simulink model "dss_test"  (Simulink 8.4)
settings: Solver=ode45  StartTime=0.0  StopTime=10.0  RelTol=1e-3
settings Model: Creator=arnaud  LastModifiedBy=arnaud

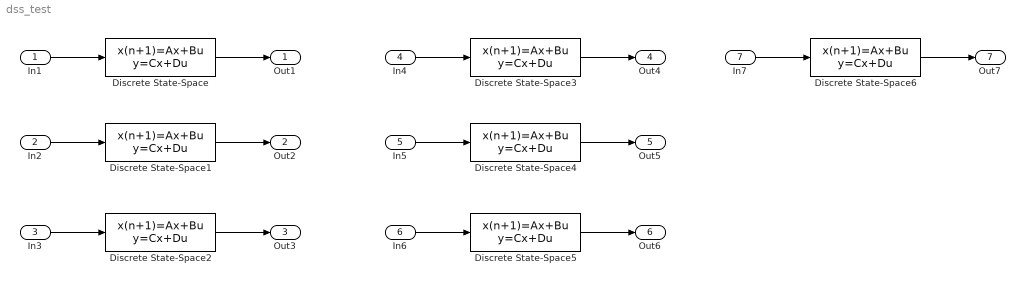
== system dss_test ==
  In1 : Inport
  In2 : Inport  Port=2
  In3 : Inport  Port=3
  In4 : Inport  Port=4
  In5 : Inport  Port=5
  In6 : Inport  Port=6
  In7 : Inport  Port=7
  Discrete State-Space : DiscreteStateSpace
  Discrete State-Space1 : DiscreteStateSpace  A=[]  B=[]  C=[]  X0=2.5
  Discrete State-Space2 : DiscreteStateSpace  A=[]  B=[]  C=[]  X0=[]
  Discrete State-Space3 : DiscreteStateSpace  A=[1 2 3; 4 5 6; 7 8 9]  B=[10 11; 12 13; 14 15]  C=[16 17 18; 19 20 21]  D=[22 23; 24 25]  X0=[]
  Discrete State-Space4 : DiscreteStateSpace  A=[1 2 3; 4 5 6; 7 8 9]  B=[10 11; 12 13; 14 15]  C=[16 17 18; 19 20 21]  D=[22 23; 24 25]  X0=[-1]
  Discrete State-Space5 : DiscreteStateSpace  A=[1 2 3; 4 5 6; 7 8 9]  B=[10 11; 12 13; 14 15]  C=[16 17 18; 19 20 21]  D=[22 23; 24 25]  X0=[-1 -2 -3]
  Discrete State-Space6 : DiscreteStateSpace  A=[1 2; 3 4]  B=[5;6]  C=[7 8]  D=9  X0=-25
  Out1 : Outport
  Out2 : Outport  Port=2
  Out3 : Outport  Port=3
  Out4 : Outport  Port=4
  Out5 : Outport  Port=5
  Out6 : Outport  Port=6
  Out7 : Outport  Port=7
  wires:
  In1/1 -> Discrete State-Space/1
  Discrete State-Space/1 -> Out1/1
  In2/1 -> Discrete State-Space1/1
  Discrete State-Space1/1 -> Out2/1
  In3/1 -> Discrete State-Space2/1
  Discrete State-Space2/1 -> Out3/1
  In4/1 -> Discrete State-Space3/1
  Discrete State-Space3/1 -> Out4/1
  In5/1 -> Discrete State-Space4/1
  Discrete State-Space4/1 -> Out5/1
  In6/1 -> Discrete State-Space5/1
  Discrete State-Space5/1 -> Out6/1
  In7/1 -> Discrete State-Space6/1
  Discrete State-Space6/1 -> Out7/1
